simulink model "elen110lab5"  (R2025b)
settings: Solver=VariableStepAuto  StartTime=0.0  StopTime=2  RelTol=1e-3

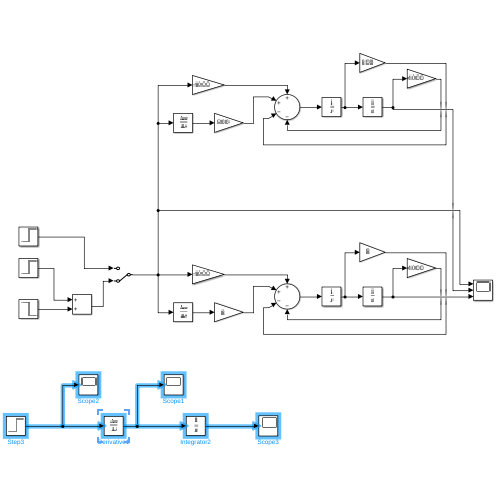
[thumbnail: Simulink's stored preview of the top-level diagram]
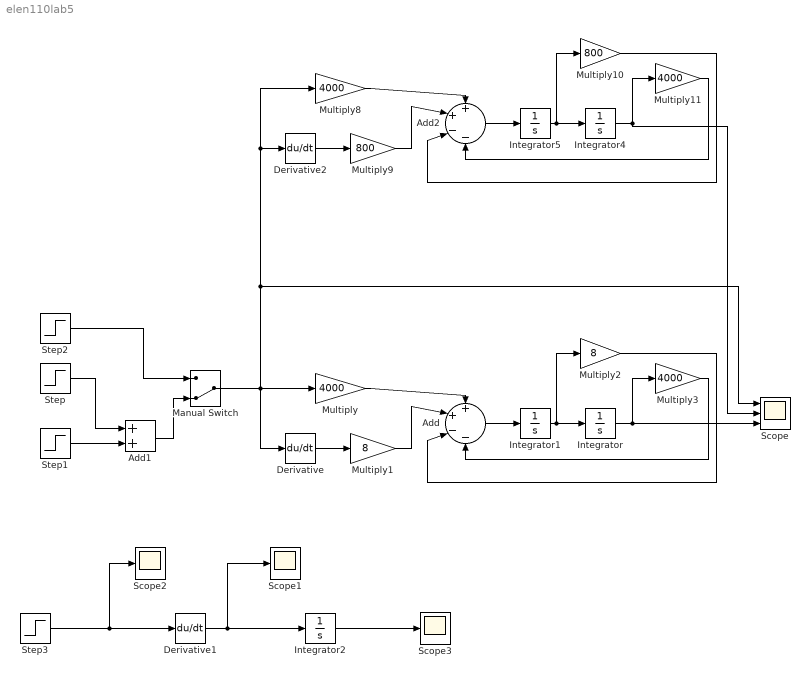
== system elen110lab5 ==
  Add : Sum  Inputs=++--
  Add1 : Sum
  Add2 : Sum  Inputs=++--
  Derivative : Derivative
  Derivative1 : Derivative
  Derivative2 : Derivative
  Integrator{,1..2,4..5} (5 alike) : Integrator
  Manual Switch : ManualSwitch  CurrentSetting=0
  Multiply{,3,8,11} (4 alike) : Gain  Gain=4000
  Multiply1 : Gain  Gain=8
  Multiply10 : Gain  Gain=800
  Multiply2 : Gain  Gain=8
  Multiply9 : Gain  Gain=800
  Scope : Scope  NumInputPorts=3
      settings: ActiveDisplayYMinimum=-0.20940457096062429  ActiveDisplayYMaximum=0.073209071231629189
  Scope1 : Scope
      settings: ActiveDisplayYMinimum=-6.597069766655998E+12  ActiveDisplayYMaximum=5.9373627899904E+13  DataLoggingVariableName=ScopeData3
  Scope2 : Scope
      settings: ActiveDisplayYMinimum=-0.37499999999999989  ActiveDisplayYMaximum=3.375
  Scope3 : Scope
      settings: ActiveDisplayYMinimum=-0.010681152343750002  ActiveDisplayYMaximum=0.096130371093750028  DataLoggingVariableName=ScopeData2
  Step : Step  Time=.2  After=.1  SampleTime=0
  Step1 : Step  Time=0  After=-.1  SampleTime=0
  Step2 : Step  After=.1  SampleTime=0
  Step3 : Step  Time=5  After=3  SampleTime=0
  wires:
  Multiply/1 -> Add/1
  Integrator1/1 -> Integrator/1, Multiply2/1
  Derivative/1 -> Multiply1/1
  Multiply1/1 -> Add/2
  Add/1 -> Integrator1/1
  Multiply2/1 -> Add/3
  Integrator/1 -> Multiply3/1, Scope/3
  Multiply3/1 -> Add/4
  Add2/1 -> Integrator5/1
  Manual Switch/1 -> Multiply8/1, Derivative2/1, Scope/1, Multiply/1, Derivative/1
  Multiply8/1 -> Add2/1
  Multiply10/1 -> Add2/3
  Integrator5/1 -> Integrator4/1, Multiply10/1
  Multiply11/1 -> Add2/4
  Derivative2/1 -> Multiply9/1
  Multiply9/1 -> Add2/2
  Integrator4/1 -> Scope/2, Multiply11/1
  Step/1 -> Add1/1
  Step1/1 -> Add1/2
  Add1/1 -> Manual Switch/2
  Step2/1 -> Manual Switch/1
  Derivative1/1 -> Scope1/1, Integrator2/1
  Integrator2/1 -> Scope3/1
  Step3/1 -> Scope2/1, Derivative1/1
